simulink model "sampleModel1452"  (R2023a)
settings: Solver=VariableStepAuto  StartTime=0.0  StopTime=10.0  RelTol=1e-3
libraries: hdlsllib x6, simulink x3
settings Model: Creator=user1  LastModifiedBy=user1

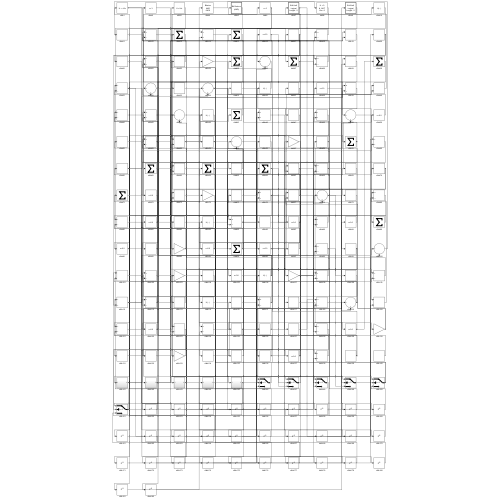
[thumbnail: Simulink's stored preview of the top-level diagram]
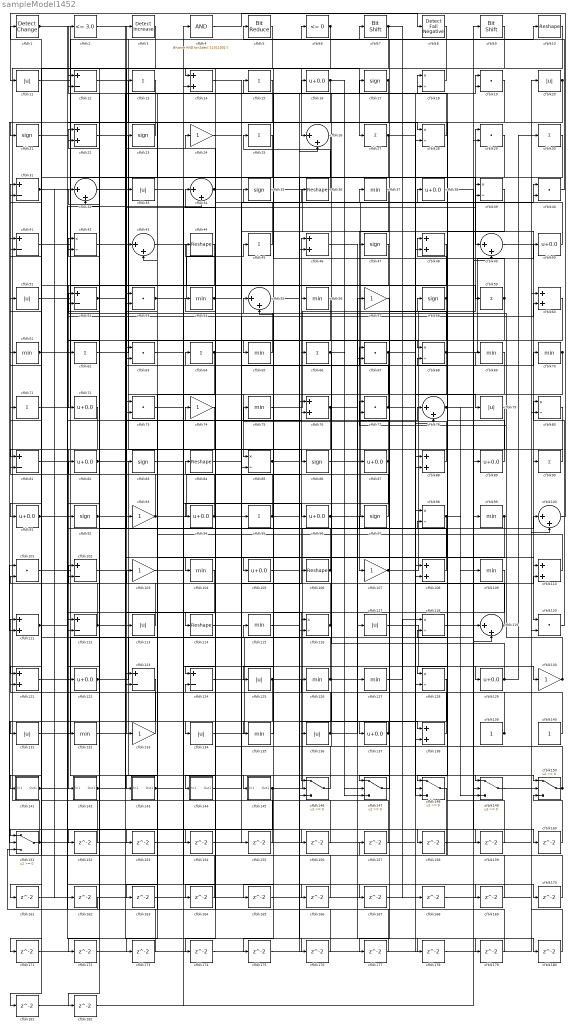
== system sampleModel1452 ==
  cfblk1 : simulink/Logic and Bit Operations/Detect Change  vinit=0  OutDataTypeStr=boolean
      settings: LibrarySourceBlock=|
      | hdlsllib/Logic and Bit
      | Operations/Detect
      | Change
  cfblk{10,36,44,84,106,114} (6 alike) : Reshape
  cfblk{26,32,34,43,49,55,78,100,119} (9 alike) : Sum  Inputs=|++
  cfblk{19,29,40,53,63,67,73,77,101,120} (10 alike) : DotProduct  OutDataTypeStr=Inherit: Inherit via internal rule
  cfblk{12,31,41,52,81,102,112,123..124} (9 alike) : Sum  Inputs=+-
  cfblk{24,57,74,93,103,107,130,133} (8 alike) : Gain
  cfblk{37,54,56,61,65,69..70,75,99,104,109,115,126..127,132,135} (16 alike) : MinMax
  cfblk{16,38,50,72,82,87,89,91,94,96,105,122,129,137} (14 alike) : Bias  Bias=0.0  SaturateOnIntegerOverflow=off
  cfblk{14,22,46,48,60,76,88,108,110..111,121,138} (12 alike) : Sum
  cfblk{11,20,33,51,79,113,117,125,131,134,136} (11 alike) : Abs  SaturateOnIntegerOverflow=off
  cfblk{18,28,39,42,68,80,85,98,116,118,128} (11 alike) : Product  Inputs=*/  RndMeth=Zero  SaturateOnIntegerOverflow=on
  cfblk{13,15,25,27,30,45,59,62,64,66,71,90,95} (13 alike) : Sum  Inputs=+
  cfblk139 : Constant  SampleTime=-1
  cfblk140 : Constant  SampleTime=-1
  cfblk141 : Subsystem
      settings: LibrarySourceBlock=|
      | hdlsllib/Ports &
      | Subsystems/Subsystem
  cfblk142 : Subsystem
      settings: LibrarySourceBlock=|
      | hdlsllib/Ports &
      | Subsystems/Subsystem
  cfblk143 : Subsystem
      settings: LibrarySourceBlock=|
      | hdlsllib/Ports &
      | Subsystems/Subsystem
  cfblk144 : Subsystem
      settings: LibrarySourceBlock=|
      | hdlsllib/Ports &
      | Subsystems/Subsystem
  cfblk145 : Subsystem
      settings: LibrarySourceBlock=|
      | hdlsllib/Ports &
      | Subsystems/Subsystem
  cfblk{146..151} (6 alike) : Switch  SaturateOnIntegerOverflow=off  InputSameDT=off
  cfblk{152..182} (31 alike) : Delay  SampleTime=1
  cfblk{17,21,23,35,47,58,83,86,92,97} (10 alike) : Signum
  cfblk2 : hdlsllib/Logic and Bit Operations/Compare To Constant  relop=<=  const=3.0  OutDataTypeStr=boolean
  cfblk3 : simulink/Logic and Bit Operations/Detect Increase  vinit=0.0  OutDataTypeStr=boolean
      settings: LibrarySourceBlock=|
      | hdlsllib/Logic and Bit
      | Operations/Detect
      | Increase
  cfblk4 : simulink/Logic and Bit Operations/Bitwise Operator  logicop=AND  UseBitMask=on  BitMask=bin2dec('11011001')  BitMaskRealWorld=Stored Integer
      settings: LibrarySourceBlock=|
      | hdlsllib/Logic and Bit
      | Operations/Bitwise
      | Operator
  cfblk5 : hdlsllib/Logic and Bit Operations/Bit Reduce  mode=AND
  cfblk6 : hdlsllib/Logic and Bit Operations/Compare To Zero  relop=<=  OutDataTypeStr=boolean
  cfblk7 : hdlsllib/Logic and Bit Operations/Bit Shift  mode=Shift Left Logical  N=0
  cfblk8 : hdlsllib/Logic and Bit Operations/Detect Fall Negative  vinit=0  OutDataTypeStr=boolean
  cfblk9 : hdlsllib/Logic and Bit Operations/Bit Shift  mode=Shift Left Logical  N=0
  wires:
  cfblk11/1 -> cfblk150/1
  cfblk74/1 -> cfblk142/1(In1)
  cfblk127/1 -> cfblk118/1
  cfblk22/1 -> cfblk134/1
  cfblk129/1 -> cfblk30/1, cfblk36/1
  cfblk151/1 -> cfblk27/1, cfblk76/1
  cfblk95/1 -> cfblk31/1, cfblk18/1
  cfblk135/1 -> cfblk55/1
  cfblk122/1 -> cfblk115/1, cfblk12/2
  cfblk90/1 -> cfblk81/1
  cfblk126/1 -> cfblk31/2, cfblk98/2
  cfblk40/1 -> cfblk5/1
  cfblk62/1 -> cfblk6/1
  cfblk100/1 -> cfblk11/1
  cfblk7/1 -> cfblk65/1, cfblk168/1
  cfblk150/1 -> cfblk84/1, cfblk126/1
  cfblk49/1 -> cfblk120/1
  cfblk23/1 -> cfblk21/1
  cfblk108/1 -> cfblk3/1
  cfblk94/1 -> cfblk61/1, cfblk56/1
  cfblk91/1 -> cfblk51/1, cfblk176/1
  cfblk123/1 -> cfblk131/1
  cfblk113/1 -> cfblk71/1
  cfblk75/1 -> cfblk58/1
  cfblk99/1 -> cfblk173/1, cfblk174/1
  cfblk36/1 -> cfblk25/1
  cfblk102/1 -> cfblk149/1
  cfblk96/1 -> cfblk40/1, cfblk178/1
  cfblk45/1 -> cfblk35/1
  cfblk70/1 -> cfblk124/1, cfblk85/2
  cfblk145/1(Out1) -> cfblk100/1, cfblk181/1
  cfblk101/1 -> cfblk146/1
  cfblk107/1 -> cfblk29/1, cfblk19/2, cfblk110/2
  cfblk33/1 -> cfblk116/1
  cfblk133/1 -> cfblk82/1
  cfblk82/1 -> cfblk145/1(In1), cfblk32/2
  cfblk67/1 -> cfblk85/1, cfblk79/1
  cfblk88/1 -> cfblk75/1
  cfblk37/1 -> cfblk107/1
  cfblk30/1 -> cfblk116/2
  cfblk119/1 -> cfblk46/1, cfblk103/1
  cfblk134/1 -> cfblk108/1
  cfblk71/1 -> cfblk10/1
  cfblk44/1 -> cfblk91/1
  cfblk87/1 -> cfblk13/1, cfblk7/1, cfblk164/1, cfblk165/1
  cfblk10/1 -> cfblk133/1
  cfblk125/1 -> cfblk9/1, cfblk151/2
  cfblk117/1 -> cfblk130/1
  cfblk140/1 -> cfblk102/1
  cfblk85/1 -> cfblk38/1, cfblk159/1
  cfblk136/1 -> cfblk57/1, cfblk64/1
  cfblk15/1 -> cfblk104/1
  cfblk53/1 -> cfblk45/1, cfblk39/2
  cfblk20/1 -> cfblk148/1, cfblk148/3
  cfblk149/1 -> cfblk20/1
  cfblk124/1 -> cfblk89/1
  cfblk114/1 -> cfblk106/1
  cfblk66/1 -> cfblk136/1, cfblk87/1
  cfblk138/1 -> cfblk111/1
  cfblk34/1 -> cfblk47/1, cfblk110/1
  cfblk92/1 -> cfblk32/1, cfblk18/2
  cfblk6/1 -> cfblk121/1, cfblk92/1
  cfblk2/1 -> cfblk68/1
  cfblk93/1 -> cfblk66/1, cfblk22/1
  cfblk42/1 -> cfblk86/1
  cfblk58/1 -> cfblk48/1, cfblk123/2
  cfblk64/1 -> cfblk95/1, cfblk163/1
  cfblk147/1 -> cfblk67/1
  cfblk104/1 -> cfblk123/1
  cfblk47/1 -> cfblk72/1
  cfblk60/1 -> cfblk93/1
  cfblk18/1 -> cfblk14/1
  cfblk35/1 -> cfblk90/1
  cfblk1/1 -> cfblk49/1, cfblk28/2
  cfblk146/1 -> cfblk54/1
  cfblk16/1 -> cfblk83/1, cfblk147/2
  cfblk118/1 -> cfblk119/2
  cfblk72/1 -> cfblk112/2
  cfblk111/1 -> cfblk34/2, cfblk74/1
  cfblk48/1 -> cfblk125/1
  cfblk144/1(Out1) -> cfblk70/1
  cfblk98/1 -> cfblk143/1(In1), cfblk149/3
  cfblk131/1 -> cfblk108/2
  cfblk54/1 -> cfblk144/1(In1), cfblk40/2
  cfblk141/1(Out1) -> cfblk97/1, cfblk167/1
  cfblk69/1 -> cfblk137/1
  cfblk12/1 -> cfblk28/1
  cfblk105/1 -> cfblk138/1
  cfblk77/1 -> cfblk63/1, cfblk78/2
  cfblk78/1 -> cfblk99/1, cfblk109/1
  cfblk97/1 -> cfblk41/1
  cfblk68/1 -> cfblk50/1, cfblk128/2, cfblk37/1
  cfblk9/1 -> cfblk26/1
  cfblk26/1 -> cfblk53/1
  cfblk61/1 -> cfblk60/2, cfblk158/1
  cfblk17/1 -> cfblk62/1, cfblk33/1, cfblk111/2
  cfblk3/1 -> cfblk102/2
  cfblk112/1 -> cfblk101/2, cfblk19/1
  cfblk39/1 -> cfblk128/1
  cfblk120/1 -> cfblk80/1
  cfblk84/1 -> cfblk69/1
  cfblk143/1(Out1) -> cfblk73/1, cfblk156/1
  cfblk116/1 -> cfblk16/1, cfblk42/2
  cfblk5/1 -> cfblk114/1
  cfblk65/1 -> cfblk24/1
  cfblk31/1 -> cfblk67/2, cfblk162/1
  cfblk28/1 -> cfblk2/1
  cfblk56/1 -> cfblk135/1
  cfblk81/1 -> cfblk113/1
  cfblk13/1 -> cfblk141/1(In1)
  cfblk86/1 -> cfblk78/1
  cfblk41/1 -> cfblk63/2
  cfblk121/1 -> cfblk43/1
  cfblk29/1 -> cfblk151/1
  cfblk25/1 -> cfblk122/1
  cfblk83/1 -> cfblk96/1
  cfblk110/1 -> cfblk73/2
  cfblk76/1 -> cfblk147/3, cfblk170/1, cfblk171/1
  cfblk132/1 -> cfblk149/2
  cfblk24/1 -> cfblk148/2
  cfblk51/1 -> cfblk59/1
  cfblk52/1 -> cfblk105/1, cfblk152/1
  cfblk130/1 -> cfblk52/1, cfblk77/2
  cfblk50/1 -> cfblk23/1
  cfblk73/1 -> cfblk14/2
  cfblk80/1 -> cfblk88/2
  cfblk89/1 -> cfblk12/1
  cfblk46/1 -> cfblk117/1
  cfblk43/1 -> cfblk127/1
  cfblk27/1 -> cfblk98/1, cfblk94/1
  cfblk103/1 -> cfblk129/1
  cfblk4/1 -> cfblk8/1
  cfblk106/1 -> cfblk42/1, cfblk22/2, cfblk44/1
  cfblk59/1 -> cfblk15/1, cfblk177/1
  cfblk57/1 -> cfblk147/1
  cfblk137/1 -> cfblk17/1, cfblk132/1
  cfblk142/1(Out1) -> cfblk39/1, cfblk76/2
  cfblk139/1 -> cfblk55/2, cfblk77/1
  cfblk152/1 -> cfblk121/2
  cfblk21/1 -> cfblk153/1
  cfblk153/1 -> cfblk48/2
  cfblk128/1 -> cfblk154/1
  cfblk154/1 -> cfblk88/1
  cfblk14/1 -> cfblk155/1
  cfblk155/1 -> cfblk81/2
  cfblk156/1 -> cfblk43/2
  cfblk148/1 -> cfblk157/1
  cfblk157/1 -> cfblk124/2
  cfblk158/1 -> cfblk100/2
  cfblk159/1 -> cfblk118/2
  cfblk38/1 -> cfblk160/1
  cfblk160/1 -> cfblk150/3
  cfblk79/1 -> cfblk161/1
  cfblk161/1 -> cfblk119/1
  cfblk162/1 -> cfblk151/3
  cfblk163/1 -> cfblk26/2
  cfblk164/1 -> cfblk1/1
  cfblk165/1 -> cfblk146/3
  cfblk63/1 -> cfblk166/1
  cfblk166/1 -> cfblk41/2
  cfblk167/1 -> cfblk60/1
  cfblk168/1 -> cfblk80/2
  cfblk55/1 -> cfblk169/1
  cfblk169/1 -> cfblk101/1
  cfblk170/1 -> cfblk68/2
  cfblk171/1 -> cfblk29/2
  cfblk19/1 -> cfblk172/1
  cfblk172/1 -> cfblk46/2
  cfblk173/1 -> cfblk112/1
  cfblk174/1 -> cfblk146/2
  cfblk109/1 -> cfblk175/1
  cfblk175/1 -> cfblk138/2
  cfblk176/1 -> cfblk34/1
  cfblk177/1 -> cfblk52/2
  cfblk178/1 -> cfblk120/2
  cfblk115/1 -> cfblk179/1
  cfblk179/1 -> cfblk53/2
  cfblk32/1 -> cfblk180/1
  cfblk180/1 -> cfblk150/2
  cfblk181/1 -> cfblk49/2
  cfblk8/1 -> cfblk182/1
  cfblk182/1 -> cfblk4/1

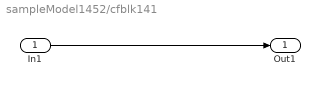
== system sampleModel1452/cfblk141 ==
  In1 : Inport
  Out1 : Outport
  wires:
  In1/1 -> Out1/1

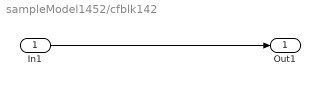
== system sampleModel1452/cfblk142 ==
  In1 : Inport
  Out1 : Outport
  wires:
  In1/1 -> Out1/1

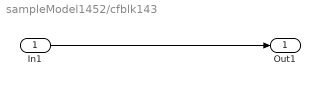
== system sampleModel1452/cfblk143 ==
  In1 : Inport
  Out1 : Outport
  wires:
  In1/1 -> Out1/1

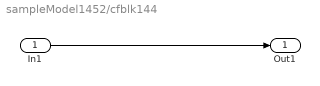
== system sampleModel1452/cfblk144 ==
  In1 : Inport
  Out1 : Outport
  wires:
  In1/1 -> Out1/1

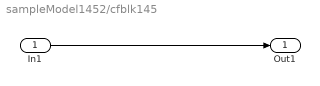
== system sampleModel1452/cfblk145 ==
  In1 : Inport
  Out1 : Outport
  wires:
  In1/1 -> Out1/1
